simulink model "FrequencyResponseTest"  (R2014a)
settings: Solver=ode3  SolverMode=SingleTasking  StartTime=0.0  StopTime=10.0  RelTol=1e-3
libraries: arduinolib x3
settings Model: ExtModeTrigDuration=2  Creator=beaverl  LastModifiedBy=beaverl
settings OptimizationCC: OptimizeModelRefInitCode=on  LifeSpan=1
settings DebuggingCC: UnderspecifiedInitializationDetection=Classic  SolverPrmCheckMsg=none
settings HardwareCC: ProdBitPerInt=16  ProdBitPerPointer=8  ProdIntDivRoundTo=Zero  ProdEndianess=LittleEndian  ProdWordSize=8  ProdHWDeviceType=Atmel->AVR
settings RTWCC: SystemTargetFile=realtime.tlc  GenerateMakefile=off  TemplateMakefile=realtime.tmf  Description=Run on Target Hardware  RTWVerbose=off  ProcessScript=realtime_make_rtw_hook
settings STFCustomTargetCC: TargetLibSuffix=.a  GenerateSampleERTMain=on  ConcurrentExecutionCompliant=off  GeneratePreprocessorConditionals=Use local settings  ERTCustomFileBanners=on  SupportNonInlinedSFcns=off  SupportVariableSizeSignals=on  MATLABClassNameForMDSCustomization=Simulink.SoftwareTarget.ERTCustomization  GRTInterface=off  SystemTargetFile=realtime.tlc
settings ERTTargetCC: CombineOutputUpdateFcns=off  SupportContinuousTime=on  SupportVariableSizeSignals=on  ExtModeTransport=3  ExtModeMexFile=ext_serial_win32_comm  ExtModeMexArgs=0 1 9600  ERTSrcFileBannerTemplate=realtime_code_template.cgt  ERTHdrFileBannerTemplate=realtime_code_template.cgt  ERTDataSrcFileTemplate=realtime_code_template.cgt  ERTDataHdrFileTemplate=realtime_code_template.cgt  ERTCustomFileTemplate=realtime_file_process.tlc

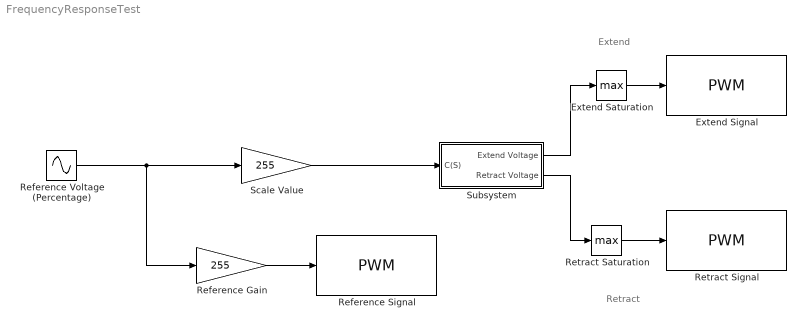
== system FrequencyResponseTest ==
  note: Retract
  note: Extend
  Extend Saturation : MinMax  Function=max  OutMin=[0]  OutMax=[255]  OutDataTypeStr=int16  SaturateOnIntegerOverflow=on
  Extend Signal : arduinolib/PWM  pinNumber=5
  Reference Gain : Gain  Gain=255
  Reference Signal : arduinolib/PWM  pinNumber=9
  Reference Voltage (Percentage) : Sin  Frequency=7  SampleTime=0
  Retract Saturation : MinMax  Function=max  OutMin=[0]  OutMax=[255]  OutDataTypeStr=int16  SaturateOnIntegerOverflow=on
  Retract Signal : arduinolib/PWM  pinNumber=7
  Scale Value : Gain  Gain=255
  Subsystem : Subsystem
  wires:
  Extend Saturation/1 -> Extend Signal/1
  Retract Saturation/1 -> Retract Signal/1
  Reference Voltage (Percentage)/1 -> Reference Gain/1, Scale Value/1
  Subsystem/1(Extend Voltage) -> Extend Saturation/1
  Subsystem/2(Retract Voltage) -> Retract Saturation/1
  Reference Gain/1 -> Reference Signal/1
  Scale Value/1 -> Subsystem/1(C(S))

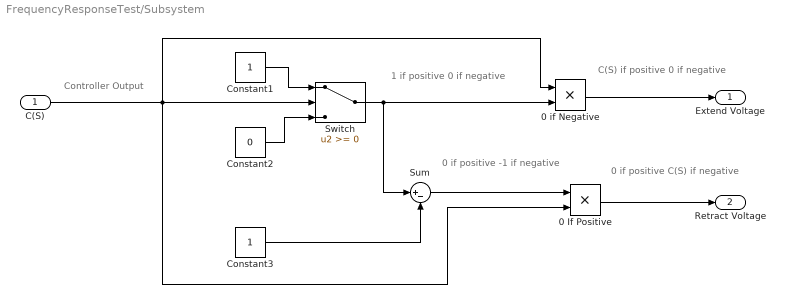
== system FrequencyResponseTest/Subsystem ==
  note: Controller Output
  note: 0 if positive
      | C(S) if negative
  note: C(S) if positive
      | 0 if negative
  note: 0 if positive
      | -1 if negative
  note: 1 if positive
      | 0 if negative
  C(S) : Inport
  0 If Positive : Product
  0 if Negative : Product
  Constant1 : Constant
  Constant2 : Constant  Value=0
  Constant3 : Constant
  Sum : Sum  Inputs=|+-
  Switch : Switch
  Extend Voltage : Outport
  Retract Voltage : Outport  Port=2
  wires:
  Constant1/1 -> Switch/1
  Constant2/1 -> Switch/3
  Switch/1 -> 0 if Negative/2, Sum/1
  Constant3/1 -> Sum/2
  0 If Positive/1 -> Retract Voltage/1
  C(S)/1 -> 0 If Positive/2, 0 if Negative/1, Switch/2
  Sum/1 -> 0 If Positive/1
  0 if Negative/1 -> Extend Voltage/1
